simulink model "Airbag_Autosar"  (R2023a)
settings: Solver=FixedStepAuto  StartTime=0.0  StopTime=10.0  RelTol=1e-3
settings Model: Creator=gurus  LastModifiedBy=gurus
settings OptimizationCC: OptimizeBlockIOStorage=off  OptimizeDataStoreBuffers=off  BusAssignmentInplaceUpdate=off
settings DebuggingCC: SFUnexpectedBacktrackingDiag=warning  SFNoUnconditionalDefaultTransitionDiag=warning
settings HardwareCC: TargetBitPerPointer=64  TargetBitPerSizeT=64  TargetBitPerPtrDiffT=64  TargetLongLongMode=on  TargetIntDivRoundTo=Zero  TargetEndianess=LittleEndian  TargetWordSize=64  TargetHWDeviceType=MATLAB Host  ProdEqTarget=off
settings RTWCC: Description=Rapid Simulation Target  SystemTargetFile=rsim.tlc  TemplateMakefile=rsim_default_tmf  GenerateReport=on  BuildConfiguration=Debug  LaunchReport=on
settings CodeAppCC: ForceParamTrailComments=on  MATLABSourceComments=on  EnableCustomComments=on
settings RSimTargetCC: TargetLangStandard=C99 (ISO)  CombineSignalStateStructs=on  SupportVariableSizeSignals=on  OptimizeReductions=off

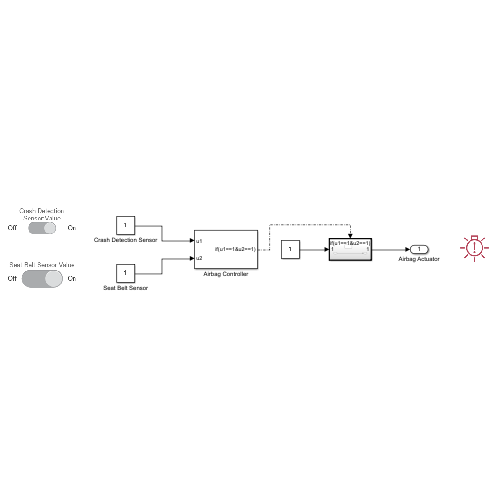
[thumbnail: Simulink's stored preview of the top-level diagram]
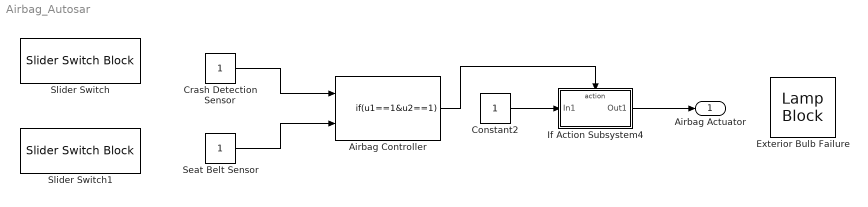
== system Airbag_Autosar ==
  Airbag Controller : If  NumInputs=2  IfExpression=u1==1&u2==1  ShowElse=off
  Constant2 : Constant
  Crash Detection Sensor : Constant
  Exterior Bulb Failure : LampBlock  LabelPosition=Hide  Icon=ExteriorBulbFailure
  If Action Subsystem4 : Subsystem  TreatAsAtomicUnit=on
  Seat Belt Sensor : Constant
  Slider Switch : SliderSwitchBlock
      settings: Values={{'Off', 'On'}, [0 1]}
  Slider Switch1 : SliderSwitchBlock
      settings: Values={{'Off', 'On'}, [0 1]}
  Airbag Actuator : Outport
  wires:
  Constant2/1 -> If Action Subsystem4/1(In1)
  Crash Detection Sensor/1 -> Airbag Controller/1
  Airbag Controller/1 -> If Action Subsystem4/Action
  Seat Belt Sensor/1 -> Airbag Controller/2
  If Action Subsystem4/1(Out1) -> Airbag Actuator/1

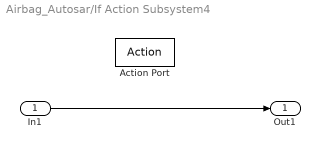
== system Airbag_Autosar/If Action Subsystem4 ==
  In1 : Inport
  Action Port : ActionPort  ActionPortLabel=if(u1==1&u2==1)
  Out1 : Outport
  wires:
  In1/1 -> Out1/1
